simulink model "Acceleration_Blocks"  (R2020b)
settings: Solver=VariableStepAuto  StartTime=0.0  StopTime=3  RelTol=1e-3
settings Model: Creator=barak  LastModifiedBy=barak

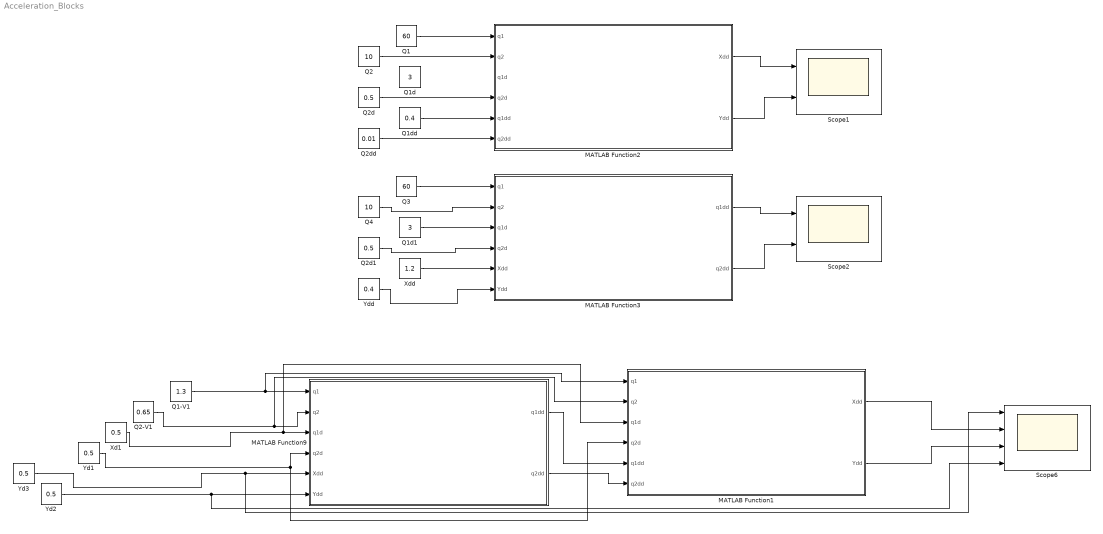
== system Acceleration_Blocks ==
  MATLAB Function1 : MATLAB Function  TreatAsAtomicUnit=on
  MATLAB Function2 : MATLAB Function  TreatAsAtomicUnit=on
  MATLAB Function3 : MATLAB Function  TreatAsAtomicUnit=on
  MATLAB Function9 : MATLAB Function  TreatAsAtomicUnit=on
  Q1 : Constant  Value=60
  Q1-V1 : Constant  Value=1.3
  Q1d : Constant  Value=3
  Q1d1 : Constant  Value=3
  Q1dd : Constant  Value=0.4
  Q2 : Constant  Value=10
  Q2-V1 : Constant  Value=0.65
  Q2d : Constant  Value=0.5
  Q2d1 : Constant  Value=0.5
  Q2dd : Constant  Value=0.01
  Q3 : Constant  Value=60
  Q4 : Constant  Value=10
  Scope1 : Scope  NumInputPorts=2
  Scope2 : Scope  NumInputPorts=2
  Scope6 : Scope  NumInputPorts=4
  Xd1 : Constant  Value=0.5
  Xdd : Constant  Value=1.2
  Yd1 : Constant  Value=0.5
  Yd2 : Constant  Value=0.5
  Yd3 : Constant  Value=0.5
  Ydd : Constant  Value=0.4
  wires:
  Q1-V1/1 -> MATLAB Function1/1(q1), MATLAB Function9/1(q1)
  Q2-V1/1 -> MATLAB Function1/2(q2), MATLAB Function9/2(q2)
  Xd1/1 -> MATLAB Function1/3(q1d), MATLAB Function9/3(q1d)
  Yd1/1 -> MATLAB Function9/4(q2d), MATLAB Function1/4(q2d)
  Yd2/1 -> Scope6/4, MATLAB Function9/6(Ydd)
  MATLAB Function1/1(Xdd) -> Scope6/2
  MATLAB Function1/2(Ydd) -> Scope6/3
  Yd3/1 -> Scope6/1, MATLAB Function9/5(Xdd)
  MATLAB Function9/1(q1dd) -> MATLAB Function1/5(q1dd)
  MATLAB Function9/2(q2dd) -> MATLAB Function1/6(q2dd)
  Q1/1 -> MATLAB Function2/1(q1)
  Q2/1 -> MATLAB Function2/2(q2)
  Q2d/1 -> MATLAB Function2/4(q2d)
  Q1dd/1 -> MATLAB Function2/5(q1dd)
  Q2dd/1 -> MATLAB Function2/6(q2dd)
  MATLAB Function2/1(Xdd) -> Scope1/1
  MATLAB Function2/2(Ydd) -> Scope1/2
  Q2d1/1 -> MATLAB Function3/4(q2d)
  Q3/1 -> MATLAB Function3/1(q1)
  Ydd/1 -> MATLAB Function3/6(Ydd)
  Xdd/1 -> MATLAB Function3/5(Xdd)
  Q4/1 -> MATLAB Function3/2(q2)
  Q1d1/1 -> MATLAB Function3/3(q1d)
  MATLAB Function3/2(q2dd) -> Scope2/2
  MATLAB Function3/1(q1dd) -> Scope2/1

== matlab function Acceleration_Blocks/MATLAB Function1 ==
  data: q1 input; q2 input; q1d input; Xdd output; q2d input; Ydd output; q1dd input; q2dd input
function [Xdd,Ydd] = RP_ACCELERATION_FW(q1,q2,q1d,q2d,q1dd,q2dd)
L1=0.5;

J = [-(L1+q2)*sind(q1),cosd(q1);
      (L1+q2)*cosd(q1),sind(q1)];
Jd = [(-(L1+q2)*cosd(q1)*q1d - sind(q1) * q2d) , -sind(q1) * q1d;
      ( (L1+q2)*sind(q1)*q1d + cosd(q1) * q2d) ,  cosd(q1) * q1d];
    
  Xdd = Jd(1,1)*q1d + Jd(1,2)*q2d + J(1,1)*q1dd + J(1,2)*q2dd;
  Ydd = Jd(2,1)*q1d + Jd(2,2)*q2d + J(2,1)*q1dd + J(2,2)*q2dd;
  
end

== matlab function Acceleration_Blocks/MATLAB Function2 ==
  data: q1 input; q2 input; q1d input; Xdd output; q2d input; Ydd output; q1dd input; q2dd input
function [Xdd,Ydd] = RP_ACCELERATION_FW(q1,q2,q1d,q2d,q1dd,q2dd)
L1=0.5;

J = [-(L1+q2)*sind(q1),cosd(q1);
      (L1+q2)*cosd(q1),sind(q1)];
Jd = [(-(L1+q2)*cosd(q1)*q1d - sind(q1) * q2d) , -sind(q1) * q1d;
      ( (L1+q2)*sind(q1)*q1d + cosd(q1) * q2d) ,  cosd(q1) * q1d];
    
  Xdd = Jd(1,1)*q1d + Jd(1,2)*q2d + J(1,1)*q1dd + J(1,2)*q2dd;
  Ydd = Jd(2,1)*q1d + Jd(2,2)*q2d + J(2,1)*q1dd + J(2,2)*q2dd;
  
end

== matlab function Acceleration_Blocks/MATLAB Function3 ==
  data: q1 input; q2 input; q1d input; q1dd output; q2d input; q2dd output; Xdd input; Ydd input
function [q1dd,q2dd] = RP_ACCELERATION_INV(q1,q2,q1d,q2d,Xdd,Ydd)
L1=0.5;

J = [-(L1+q2)*sind(q1),cosd(q1);
      (L1+q2)*cosd(q1),sind(q1)];
Jd = [(-(L1+q2)*cosd(q1)*q1d - sind(q1) * q2d) , -sind(q1) * q1d;
      ( (L1+q2)*sind(q1)*q1d + cosd(q1) * q2d) ,  cosd(q1) * q1d];
    
  Xdd = Jd(1,1)*q1d + Jd(1,2)*q2d + J(1,1)* q1dd + J(1,2) * q2dd ;
  Ydd = Jd(2,1)*q1d + Jd(2,2)*q2d + J(2,1)* q1dd + J(2,2) * q2dd ;
  
  Joint_ACC = (J^(-1)) * ( [Xdd ; Ydd] - (Jd * [q1d ; q2d] ) );
  
  q1dd = Joint_ACC(1);
  q2dd = Joint_ACC(2);
end

== matlab function Acceleration_Blocks/MATLAB Function9 ==
  data: q1 input; q2 input; q1d input; q1dd output; q2d input; q2dd output; Xdd input; Ydd input
function [q1dd,q2dd] = RP_ACCELERATION_INV(q1,q2,q1d,q2d,Xdd,Ydd)
L1=0.5;

J = [-(L1+q2)*sind(q1),cosd(q1);
      (L1+q2)*cosd(q1),sind(q1)];
Jd = [(-(L1+q2)*cosd(q1)*q1d - sind(q1) * q2d) , -sind(q1) * q1d;
      ( (L1+q2)*sind(q1)*q1d + cosd(q1) * q2d) ,  cosd(q1) * q1d];
    
  Xdd = Jd(1,1)*q1d + Jd(1,2)*q2d + J(1,1)* q1dd + J(1,2) * q2dd ;
  Ydd = Jd(2,1)*q1d + Jd(2,2)*q2d + J(2,1)* q1dd + J(2,2) * q2dd ;
  
  Joint_ACC = (J^(-1)) * ( [Xdd ; Ydd] - (Jd * [q1d ; q2d] ) );
  
  q1dd = Joint_ACC(1);
  q2dd = Joint_ACC(2);
end
